simulink model "Model_DT_statespacesystem"  (R2024b)
settings: Solver=ode45  StartTime=0.0  StopTime=5  RelTol=1e-3
values from neighbouring files (symbols this model uses):
  Ts = Ts_values(i)    [A_final_results.m]
settings Model: Creator=Riccardo Grosso  LastModifiedBy=Buton
settings DataIOCC: ReturnWorkspaceOutputs=off

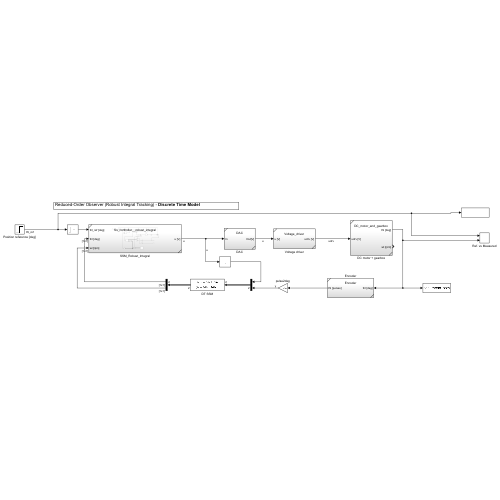
[thumbnail: Simulink's stored preview of the top-level diagram]
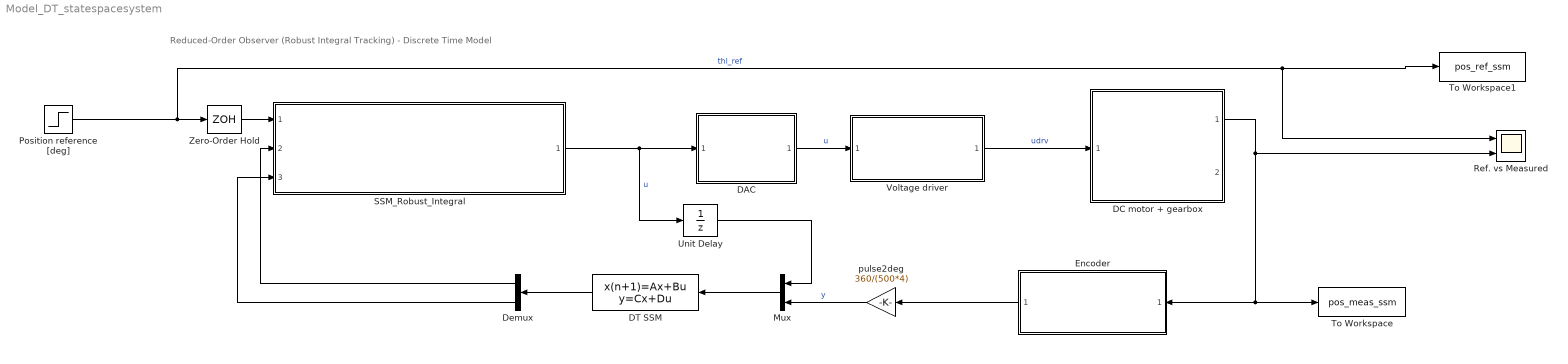
== system Model_DT_statespacesystem ==
  note: Reduced-Order Observer (Robust Integral Tracking) - Discrete Time Model
  DAC : Subsystem  ReferencedSubsystem=DAC
  DC motor + gearbox : Subsystem  ReferencedSubsystem=DC_motor_and_gearbox
  DT SSM : DiscreteStateSpace  A=-0.617518153598703  B=[4.60319591415276 -1076.4565525162]  C=[0;0.0427627704356467]  D=[0 1;0.514652948889743 28.4585767008451]  SampleTime=Ts
  Demux : Demux  Outputs=2
  Encoder : Subsystem  ReferencedSubsystem=Encoder
  Mux : Mux  Inputs=2
  Position reference [deg] : Step  Time=0  After=50  SampleTime=0
  Ref. vs Measured : Scope  NumInputPorts=2
  SSM_Robust_Integral : Subsystem  ReferencedSubsystem=Ss_controller__robust_integral
  To Workspace : ToWorkspace  VariableName=pos_meas_ssm  SaveFormat=Timeseries  SampleTime=-1
  To Workspace1 : ToWorkspace  VariableName=pos_ref_ssm  SaveFormat=Timeseries  SampleTime=-1
  Unit Delay : UnitDelay  SampleTime=-1  HasFrameUpgradeWarning=on
  Voltage driver : Subsystem  ReferencedSubsystem=Voltage_driver
  Zero-Order Hold : ZeroOrderHold  SampleTime=Ts
  pulse2deg : Gain  Gain=360/(500*4)
  wires:
  DAC/1 -> Voltage driver/1  "u"
  Voltage driver/1 -> DC motor + gearbox/1  "udrv"
  Encoder/1 -> pulse2deg/1
  DC motor + gearbox/1 -> Encoder/1, To Workspace/1, Ref. vs Measured/2
  Position reference [deg]/1 -> Zero-Order Hold/1, To Workspace1/1, Ref. vs Measured/1  "thl_ref"
  SSM_Robust_Integral/1 -> Unit Delay/1, DAC/1  "u"
  Mux/1 -> DT SSM/1
  pulse2deg/1 -> Mux/2  "y"
  Demux/1 -> SSM_Robust_Integral/2
  Demux/2 -> SSM_Robust_Integral/3
  Zero-Order Hold/1 -> SSM_Robust_Integral/1
  Unit Delay/1 -> Mux/1
  DT SSM/1 -> Demux/1
